simulink model "SingleInverterInfBus"  (R2020b)
settings: Solver=FixedStepAuto  StartTime=0.0  StopTime=20  FixedStep=Ts  RelTol=1e-3
values from neighbouring files (symbols this model uses):
  Cdc = 0.125    [Para.m]    (also in Para_VFM_FFL_Inverter.m = 0.101859163579; Para_VFM_FFL_Inverter_v2.m = 0.101859163579)
  Cf = 0.02    [Para.m]    (also in Para_VFM_FFL_Inverter.m; Para_VFM_FFL_Inverter_v2.m)
  Lc = 0.02    [Para.m]    (also in Para_VFM_FFL_Inverter.m; Para_VFM_FFL_Inverter_v2.m)
  Lf = 0.05    [Para.m]    (also in Para_VFM_FFL_Inverter.m; Para_VFM_FFL_Inverter_v2.m)
  m = 5/100    (= 0.05)    [Para.m]    (also in Para_VFM_FFL_Inverter.m; Para_VFM_FFL_Inverter_v2.m)
  Rline = Xline/5    (= 0.19)    [Para.m]    (also in Para_VFM_FFL_Inverter.m; Para_VFM_FFL_Inverter_v2.m)
  Sbase = 1    [Para.m]    (also in Para_VFM_FFL_Inverter.m; Para_VFM_FFL_Inverter_v2.m)
  Ts = 1/Fs    (= 0.0001)    [Para.m]    (also in Para_VFM_FFL_Inverter.m; Para_VFM_FFL_Inverter_v2.m = 5e-05)
  Vbase = 1    [Para.m]    (also in Para_VFM_FFL_Inverter.m; Para_VFM_FFL_Inverter_v2.m)
  vdc_ref = 2.5    [Para.m]    (also in Para_VFM_FFL_Inverter.m; Para_VFM_FFL_Inverter_v2.m)
  w_droop = 1*2*pi    (= 6.28318530718)    [Para.m]    (also in Para_VFM_FFL_Inverter.m = 31.4159265359; Para_VFM_FFL_Inverter_v2.m = 31.4159265359)
  w_i = 600*2*pi    (= 3769.91118431)    [Para.m]    (also in Para_VFM_FFL_Inverter.m; Para_VFM_FFL_Inverter_v2.m)
  w_pll = 15*2*pi    (= 94.2477796077)    [Para.m]    (also in Para_VFM_FFL_Inverter.m; Para_VFM_FFL_Inverter_v2.m)
  w_tau = 200*2*pi    (= 1256.63706144)    [Para.m]    (also in Para_VFM_FFL_Inverter.m; Para_VFM_FFL_Inverter_v2.m)
  w_v = 300*2*pi    (= 1884.95559215)    [Para.m]    (also in Para_VFM_FFL_Inverter.m; Para_VFM_FFL_Inverter_v2.m)
  w_vdc = 5*2*pi    (= 31.4159265359)    [Para.m]    (also in Para_VFM_FFL_Inverter.m; Para_VFM_FFL_Inverter_v2.m)
  Wbase = 2*pi*50    (= 314.159265359)    [Para.m]    (also in Para_VFM_FFL_Inverter.m; Para_VFM_FFL_Inverter_v2.m)
  Xline = 0.95    [Para.m]    (also in Para_VFM_FFL_Inverter.m; Para_VFM_FFL_Inverter_v2.m)
  Zbase = Vbase/Ibase    (= 1)    [Para.m]    (also in Para_VFM_FFL_Inverter.m; Para_VFM_FFL_Inverter_v2.m)
undefined symbols (not defined in the file or in its folder): DiscIntNeverNeededParam, initial
libraries: powerlib x282, SimplusGT x7
(part 1 of 8)
settings Model: Creator=admin_user  LastModifiedBy=admin_user
settings DataIOCC: ReturnWorkspaceOutputs=off

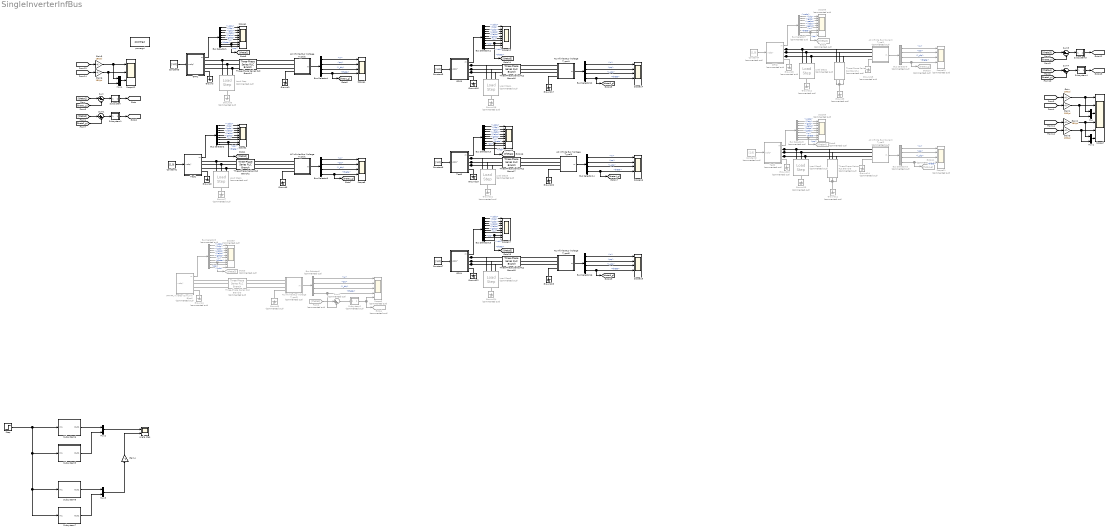
== system SingleInverterInfBus ==
  AC Infinite Bus (Current Type)1 : Subsystem  Commented=on  AncestorBlock=|  mask{Ts=Ts, Sbase=Sbase, Vbase=Vbase, Wbase=Wbase, id=1, iq=0, theta0=0, w=1}
      | SimplusGT/AC Infinite Bus
      | (Current Type)
      mask prompts: Ts "Ts (s), sampling period"; Sbase "Sbase (VA), base power"; Vbase "Vbase (V), base voltage"; Wbase "Wbase (rad/s), base angular frequency"; id "id (pu), d-axis current"; iq "iq (pu), q-axis current"; theta0 "theta0 (rad), initial angle"; w "w (pu), angular frequency"
  AC Infinite Bus (Current Type)2 : Subsystem  Commented=on  AncestorBlock=|  mask{Ts=Ts, Sbase=Sbase, Vbase=Vbase, Wbase=Wbase, id=1, iq=0, theta0=0, w=1}
      | SimplusGT/AC Infinite Bus
      | (Current Type)
      mask prompts: Ts "Ts (s), sampling period"; Sbase "Sbase (VA), base power"; Vbase "Vbase (V), base voltage"; Wbase "Wbase (rad/s), base angular frequency"; id "id (pu), d-axis current"; iq "iq (pu), q-axis current"; theta0 "theta0 (rad), initial angle"; w "w (pu), angular frequency"
  AC Infinite Bus (Voltage Type)1 : Subsystem  AncestorBlock=|  mask{Ts=Ts, Sbase=Sbase, Vbase=Vbase, Wbase=Wbase, vd=1, vq=0, theta0=0, w=Wbase*1, R=1e-30}
      | SimplusGT/AC Infinite Bus
      | (Voltage Type)
      mask prompts: Ts "Ts (s), samping period"; Sbase "Sbase (VA), power base"; Vbase "Vbase (V), voltage base"; Wbase "Wbase (rad/s), frequency base"; vd "vd (pu), d-axis voltage"; vq "vq (pu), q-axis voltage"; theta0 "theta0 (rad), initial angle"; w "w (rad/s), frequency"; R "R (Ohm), resistance"
  AC Infinite Bus (Voltage Type)2 : Subsystem  AncestorBlock=|  mask{Ts=Ts, Sbase=Sbase, Vbase=Vbase, Wbase=Wbase, vd=1, vq=0, theta0=0, w=Wbase*1, R=1e-30}
      | SimplusGT/AC Infinite Bus
      | (Voltage Type)
      mask prompts: Ts "Ts (s), samping period"; Sbase "Sbase (VA), power base"; Vbase "Vbase (V), voltage base"; Wbase "Wbase (rad/s), frequency base"; vd "vd (pu), d-axis voltage"; vq "vq (pu), q-axis voltage"; theta0 "theta0 (rad), initial angle"; w "w (rad/s), frequency"; R "R (Ohm), resistance"
  AC Infinite Bus (Voltage Type)3 : Subsystem  Commented=on  AncestorBlock=|  mask{Ts=Ts, Sbase=Sbase, Vbase=Vbase, Wbase=Wbase, vd=1, vq=0, theta0=0, w=Wbase*1, R=1e-30}
      | SimplusGT/AC Infinite Bus
      | (Voltage Type)
      mask prompts: Ts "Ts (s), samping period"; Sbase "Sbase (VA), power base"; Vbase "Vbase (V), voltage base"; Wbase "Wbase (rad/s), frequency base"; vd "vd (pu), d-axis voltage"; vq "vq (pu), q-axis voltage"; theta0 "theta0 (rad), initial angle"; w "w (rad/s), frequency"; R "R (Ohm), resistance"
  AC Infinite Bus (Voltage Type)4 : Subsystem  AncestorBlock=|  mask{Ts=Ts, Sbase=Sbase, Vbase=Vbase, Wbase=Wbase, vd=1, vq=0, theta0=0, w=Wbase*1, R=1e-30}
      | SimplusGT/AC Infinite Bus
      | (Voltage Type)
      mask prompts: Ts "Ts (s), samping period"; Sbase "Sbase (VA), power base"; Vbase "Vbase (V), voltage base"; Wbase "Wbase (rad/s), frequency base"; vd "vd (pu), d-axis voltage"; vq "vq (pu), q-axis voltage"; theta0 "theta0 (rad), initial angle"; w "w (rad/s), frequency"; R "R (Ohm), resistance"
  AC Infinite Bus (Voltage Type)5 : Subsystem  AncestorBlock=|  mask{Ts=Ts, Sbase=Sbase, Vbase=Vbase, Wbase=Wbase, vd=1, vq=0, theta0=0, w=Wbase*1, R=1e-30}
      | SimplusGT/AC Infinite Bus
      | (Voltage Type)
      mask prompts: Ts "Ts (s), samping period"; Sbase "Sbase (VA), power base"; Vbase "Vbase (V), voltage base"; Wbase "Wbase (rad/s), frequency base"; vd "vd (pu), d-axis voltage"; vq "vq (pu), q-axis voltage"; theta0 "theta0 (rad), initial angle"; w "w (rad/s), frequency"; R "R (Ohm), resistance"
  AC Infinite Bus (Voltage Type)6 : Subsystem  AncestorBlock=|  mask{Ts=Ts, Sbase=Sbase, Vbase=Vbase, Wbase=Wbase, vd=1, vq=0, theta0=0, w=Wbase*1, R=1e-30}
      | SimplusGT/AC Infinite Bus
      | (Voltage Type)
      mask prompts: Ts "Ts (s), samping period"; Sbase "Sbase (VA), power base"; Vbase "Vbase (V), voltage base"; Wbase "Wbase (rad/s), frequency base"; vd "vd (pu), d-axis voltage"; vq "vq (pu), q-axis voltage"; theta0 "theta0 (rad), initial angle"; w "w (rad/s), frequency"; R "R (Ohm), resistance"
  Angle step : Scope  NumInputPorts=2
  Bus Selector1 : BusSelector  OutputSignals=vcdq,ildq,igdq,vcabc,ilabc,igabc,w,theta,pq
  Bus Selector10 : BusSelector  Commented=on  OutputSignals=w,pq,i_dq,theta
  Bus Selector11 : BusSelector  OutputSignals=vcdq,ildq,igdq,vcabc,ilabc,igabc,w,theta,pq,vdc
  Bus Selector{4..5,12,14,16} (5 alike) : BusSelector  OutputSignals=w,pq,i_dq,theta
  Bus Selector13 : BusSelector  OutputSignals=vcdq,ildq,igdq,vcabc,ilabc,igabc,w,theta,pq,vdc
  Bus Selector15 : BusSelector  OutputSignals=vcdq,ildq,igdq,vcabc,ilabc,igabc,w,theta,pq,vdc
  Bus Selector2 : BusSelector  OutputSignals=vcdq,ildq,igdq,vcabc,ilabc,igabc,w,theta,pq
  Bus Selector3 : BusSelector  Commented=on  OutputSignals=vcdq,ildq,igdq,vcabc,ilabc,igabc,w,theta,pq,vdc
  Bus Selector6 : BusSelector  Commented=on  OutputSignals=w,pq,i_dq,theta
  Bus Selector7 : BusSelector  Commented=on  OutputSignals=vcdq,ildq,igdq,vcabc,ilabc,igabc,w,theta,pq
  Bus Selector8 : BusSelector  Commented=on  OutputSignals=vcdq,ildq,igdq,vcabc,ilabc,igabc,w,theta,pq
  Bus Selector9 : BusSelector  Commented=on  OutputSignals=w,pq,i_dq,theta
  Constant{1,3,5..7} (5 alike) : Constant  Value=[1,0]
  Constant2 : Constant  Commented=on  Value=[1,0]
  Constant4 : Constant  Commented=on  Value=[1,0]
  From2 : From  Commented=on  GotoTag=theta3
  GFM1 : Subsystem  mask{Ts=Ts, Sbase=Sbase, Vbase=Vbase, Wbase=Wbase, w_i=w_i, w_v=w_v, w_droop=w_droop, m=m, Lf=Lf, Cf=Cf, Lc=Lc}
      mask prompts: Ts "Ts (s), sampling period"; Sbase "Sbase (VA), base power"; Vbase "Vbase (V), base voltage"; Wbase "Wbase (rad/s), base frequency"; w_i "w_i (rad/s), current-loop bandwidth"; w_v "w_v (rad/s), voltage-loop bandwidth"; w_droop "w_droop (rad/s), droop bandwidth"; m "m (pu), frequency droop gain"; Lf "Lf (pu), LCL filter"; Cf "Cf (pu), LCL filter"; Lc "Lc (pu), LCL filter"
  GFM2 : Subsystem  Commented=on  mask{Ts=Ts, Sbase=Sbase, Vbase=Vbase, Wbase=Wbase, w_i=w_i, w_v=w_v, w_droop=w_droop, m=m, Lf=Lf, Cf=Cf, Lc=Lc}
      mask prompts: Ts "Ts (s), sampling period"; Sbase "Sbase (VA), base power"; Vbase "Vbase (V), base voltage"; Wbase "Wbase (rad/s), base frequency"; w_i "w_i (rad/s), current-loop bandwidth"; w_v "w_v (rad/s), voltage-loop bandwidth"; w_droop "w_droop (rad/s), droop bandwidth"; m "m (pu), frequency droop gain"; Lf "Lf (pu), LCL filter"; Cf "Cf (pu), LCL filter"; Lc "Lc (pu), LCL filter"
  GFM3 : Subsystem  mask{Ts=Ts, Sbase=Sbase, Vbase=Vbase, Wbase=Wbase, w_i=w_i, w_v=w_v, w_droop=w_droop, m=m, Lf=Lf, Cf=Cf, Lc=Lc, Cdc=Cdc, vdc_ref=vdc_ref, w_vdc=w_vdc/10}
      mask prompts: Ts "Ts (s), sampling period"; Sbase "Sbase (VA), base power"; Vbase "Vbase (V), base voltage"; Wbase "Wbase (rad/s), base frequency"; w_i "w_i (rad/s), current-loop bandwidth"; w_v "w_v (rad/s), voltage-loop bandwidth"; w_droop "w_droop (rad/s), droop bandwidth"; m "m (pu), frequency droop gain"; Lf "Lf (pu), LCL filter"; Cf "Cf (pu), LCL filter"; Lc "Lc (pu), LCL filter"
  GFM4 : Subsystem  mask{Ts=Ts, Sbase=Sbase, Vbase=Vbase, Wbase=Wbase, w_i=w_i, w_v=w_v, w_droop=w_droop, m=m, Lf=Lf, Cf=Cf, Lc=Lc, Cdc=Cdc, vdc_ref=vdc_ref, w_vdc=w_vdc/1}
      mask prompts: Ts "Ts (s), sampling period"; Sbase "Sbase (VA), base power"; Vbase "Vbase (V), base voltage"; Wbase "Wbase (rad/s), base frequency"; w_i "w_i (rad/s), current-loop bandwidth"; w_v "w_v (rad/s), voltage-loop bandwidth"; w_droop "w_droop (rad/s), droop bandwidth"; m "m (pu), frequency droop gain"; Lf "Lf (pu), LCL filter"; Cf "Cf (pu), LCL filter"; Lc "Lc (pu), LCL filter"
  Gain{,1..3,5..6} (6 alike) : Gain  Gain=180/pi
  Gain4 : Gain  Gain=-1
  Goto10 : Goto  Commented=on  GotoTag=theta3_g
  Goto11 : Goto  Commented=on  GotoTag=theta4_g
  Goto3 : Goto  Commented=on  GotoTag=theta3
  Goto4 : Goto  Commented=on  GotoTag=theta_diff3
  Goto8 : Goto  Commented=on  GotoTag=theta4
  Goto9 : Goto  Commented=on  GotoTag=theta3
  Ground{,1..3,16..17,19..20,22..23} (10 alike) : powerlib/Elements/Ground  LConnTagsString=a
  Ground{4..15,18,21,24} (15 alike) : powerlib/Elements/Ground  Commented=on  LConnTagsString=a
  Load Step{,1,4..6} (5 alike) : SimplusGT/Load Step  Commented=on  t0=0  R=4*Zbase  Reverse=0
      settings: SourceProductName=Simplus Grid Tool
  Load Step2 : SimplusGT/Load Step  Commented=on  t0=0  R=3*Zbase  Reverse=0
      settings: SourceProductName=Simplus Grid Tool
  Load Step3 : SimplusGT/Load Step  Commented=on  t0=0  R=3*Zbase  Reverse=0
      settings: SourceProductName=Simplus Grid Tool
  Mux{,1..4} (5 alike) : Mux  Inputs=2
  Scope1 : Scope  NumInputPorts=9
  Scope10 : Scope  Commented=on  NumInputPorts=5
  Scope11 : Scope  Commented=on  NumInputPorts=5
  Scope12 : Scope  NumInputPorts=3
  Scope13 : Scope  NumInputPorts=10
  Scope{4..5,14,16,18} (5 alike) : Scope  NumInputPorts=5
  Scope15 : Scope  NumInputPorts=10
  Scope17 : Scope  NumInputPorts=10
  Scope2 : Scope  NumInputPorts=9
  Scope3 : Scope  Commented=on  NumInputPorts=10
  Scope6 : Scope  Commented=on  NumInputPorts=5
  Scope7 : Scope  NumInputPorts=6
  Scope8 : Scope  Commented=on  NumInputPorts=9
  Scope9 : Scope  Commented=on  NumInputPorts=9
  Step : Step  Time=3  After=-1  SampleTime=0
  Subsystem : Subsystem
  Subsystem1 : Subsystem
  Subsystem2 : Subsystem  Commented=on
  Subsystem3 : Subsystem
  Subsystem4 : Subsystem
  Subsystem5 : Subsystem  mask{kp=1*2*pi, ki=1*2*pi*2.5*2*pi}
  Subsystem6 : Subsystem  mask{kd=1/(2.5*2*pi), ki=1*2*pi*2.5*2*pi}
  Subsystem7 : Subsystem  mask{kp=1*2*pi, ki=1*2*pi*2.5*2*pi}
  Subsystem8 : Subsystem  mask{kd=1/(2.5*2*pi), ki=1*2*pi*2.5*2*pi}
  Sum{,1,3..4} (4 alike) : Sum  Inputs=|+-
  Sum2 : Sum  Commented=on  Inputs=|+-
  Test1 : Subsystem  mask{Ts=Ts, Sbase=Sbase, Vbase=Vbase, Wbase=Wbase, w_i=w_i*1, w_v=w_v, w_pll=w_pll, w_tau=w_tau, m=m, Lf=Lf, Cf=Cf, Lc=Lc}
      mask prompts: Ts "Ts (s), sampling period"; Sbase "Sbase (VA), base power"; Vbase "Vbase (V), base voltage"; Wbase "Wbase (rad/s), base frequency"; w_i "w_i (rad/s), current-loop bandwidth"; w_v "w_v (rad/s), voltage-loop bandwidth"; w_pll "w_pll (rad/s), PLL bandwidth"; w_tau "w_tau (rad/s), pll LPF bandwidth"; m "m (pu), frequency droop gain"; Lf "Lf (pu), LCL filter"; Cf "Cf (pu), LCL filter"; Lc "Lc (pu), LCL filter"
  Test2 : Subsystem  Commented=on  mask{Ts=Ts, Sbase=Sbase, Vbase=Vbase, Wbase=Wbase, w_i=w_i, w_v=w_v, w_pll=w_pll, w_tau=w_tau, m=m, Lf=Lf, Cf=Cf, Lc=Lc}
      mask prompts: Ts "Ts (s), sampling period"; Sbase "Sbase (VA), base power"; Vbase "Vbase (V), base voltage"; Wbase "Wbase (rad/s), base frequency"; w_i "w_i (rad/s), current-loop bandwidth"; w_v "w_v (rad/s), voltage-loop bandwidth"; w_pll "w_pll (rad/s), PLL bandwidth"; w_tau "w_tau (rad/s), pll LPF bandwidth"; m "m (pu), frequency droop gain"; Lf "Lf (pu), LCL filter"; Cf "Cf (pu), LCL filter"; Lc "Lc (pu), LCL filter"
  Test3 : Subsystem  mask{Ts=Ts, Sbase=Sbase, Vbase=Vbase, Wbase=Wbase, w_i=w_i*1, w_v=w_v, w_pll=w_pll, w_tau=w_tau, m=m, Lf=Lf, Cf=Cf, Lc=Lc, Cdc=Cdc, vdc_ref=vdc_ref, w_vdc=w_vdc/10}
      mask prompts: Ts "Ts (s), sampling period"; Sbase "Sbase (VA), base power"; Vbase "Vbase (V), base voltage"; Wbase "Wbase (rad/s), base frequency"; w_i "w_i (rad/s), current-loop bandwidth"; w_v "w_v (rad/s), voltage-loop bandwidth"; w_pll "w_pll (rad/s), PLL bandwidth"; w_tau "w_tau (rad/s), pll LPF bandwidth"; m "m (pu), frequency droop gain"; Lf "Lf (pu), LCL filter"; Cf "Cf (pu), LCL filter"; Lc "Lc (pu), LCL filter"
  Three-Phase Series RLC Branch{1..2,6..8} (5 alike) : powerlib/Elements/Three-Phase Series RLC Branch  LConnTagsString=A|B|C  RConnTagsString=A|B|C  BranchType=RL  Resistance=Rline*Zbase  Inductance=Xline*Zbase/Wbase  Capacitance=1/Wbase  Measurements=None
  Three-Phase Series RLC Branch3 : powerlib/Elements/Three-Phase Series RLC Branch  Commented=on  LConnTagsString=A|B|C  RConnTagsString=A|B|C  BranchType=RL  Resistance=Rline*Zbase  Inductance=Xline*Zbase/Wbase  Capacitance=1/Wbase  Measurements=None
  Three-Phase Series RLC Branch4 : powerlib/Elements/Three-Phase Series RLC Branch  Commented=on  LConnTagsString=A|B|C  RConnTagsString=A|B|C  BranchType=RL  Resistance=Rline*Zbase  Inductance=Xline*Zbase/Wbase  Capacitance=1/Wbase  Measurements=None
  Three-Phase Series RLC Branch5 : powerlib/Elements/Three-Phase Series RLC Branch  Commented=on  LConnTagsString=A|B|C  RConnTagsString=A|B|C  BranchType=RL  Resistance=Rline*Zbase  Inductance=Xline*Zbase/Wbase  Capacitance=1/Wbase  Measurements=None
  VFM-FFL Inverter (Simulink Block) : Subsystem  Commented=on  mask{Ts=Ts, Sbase=Sbase, Vbase=Vbase, Wbase=Wbase, w_i=w_i, w_v=w_v, w_pll=w_pll, w_tau=w_tau, m=m, wLf=Lf, wCf=Cf, wLc=Lc, Cdc=Cdc, vdc_ref=vdc_ref, w_vdc=w_vdc}
      mask prompts: Ts "Ts (s), sampling period"; Sbase "Sbase (VA), base power"; Vbase "Vbase (V), base voltage"; Wbase "Wbase (rad/s), base frequency"; w_i "w_i (rad/s), current-loop bandwidth"; w_v "w_v (rad/s), voltage-loop bandwidth"; w_pll "w_pll (rad/s), PLL bandwidth"; w_tau "w_tau (rad/s), pll LPF bandwidth"; m "m (pu), frequency droop gain"; wLf "wLf (pu), LCL filter"; wCf "wCf (pu), LCL filter"; wLc "wLc (pu), LCL filter"; Cdc "Cdc (pu), dc-link capacitor"; vdc_ref "vdc_ref (pu), dc-link voltage reference"; w_vdc "w_vdc (rad/s), dc-link voltage loop bandwidth"
  powergui : powerlib/powergui  Priority=1  SimulationMode=Discrete  SampleTime=Ts  frequency=60  Iterations=50  frequencyindice=0  Pbase=100e6  ErrMax=1e-4  UnitsV=kV  UnitsW=MW  buscounter=0  FunctionMessages=off  echomessages=off  EnableUseOfTLC=off  CurrentSourceSwitches=off  DisableSnubberDevices=off  DisableRonSwitches=off  DisableVfSwitches=off  DisplayEquations=off  AutomaticDiscreteSolvers=off  SolverType=Tustin/Backward Euler (TBE)  Interpol=off  ExternalGateDelay=off  methode=off  Ts=100  x0status=blocks  SPID=on  SwTol=0  HookPort=off  NonlinearTolerance=1e-4  nMaxIteration=100  ContinueOnMaxIteration=off  RestoreLinks=warning  ResistiveCurrentMeasurement=off  Frange=[0:2:500]  Ylog=off  Xlog=on  ShowGrid=off  save=off  variable=ZData  structure=0  ZoomFFT=off  StartTime=0.0  cycles=1  DisplayStyle=1  fundamental=60  FreqAxis=off  MaxFrequency=1000  frequencyindicesteady=1  RmsSteady=1  display=off
  wires:
  Constant3/1 -> GFM1/1(vcdq*)
  Bus Selector1/7 -> Scope1/7  "<w>"
  Bus Selector1/3 -> Scope1/3  "<igdq>"
  Bus Selector1/2 -> Scope1/2  "<ildq>"
  Bus Selector1/1 -> Scope1/1  "<vcdq>"
  Bus Selector1/5 -> Scope1/5  "<ilabc>"
  Bus Selector1/6 -> Scope1/6  "<igabc>"
  Bus Selector1/4 -> Scope1/4  "<vcabc>"
  Bus Selector1/8 -> [theta1], Scope1/8  "<theta>"
  GFM1/1(m) -> Bus Selector1/1
  Test1/1(m) -> Bus Selector2/1
  Bus Selector2/8 -> Scope2/8, [theta2]  "<theta>"
  Bus Selector2/6 -> Scope2/6  "<igabc>"
  Bus Selector2/1 -> Scope2/1  "<vcdq>"
  Bus Selector2/2 -> Scope2/2  "<ildq>"
  Bus Selector2/5 -> Scope2/5  "<ilabc>"
  Bus Selector2/4 -> Scope2/4  "<vcabc>"
  Bus Selector2/3 -> Scope2/3  "<igdq>"
  Bus Selector2/7 -> Scope2/7  "<w>"
  Constant1/1 -> Test1/1(vcdq*)
  Bus Selector3/5 -> Scope3/5  "<ilabc>"
  Bus Selector3/2 -> Scope3/2  "<ildq>"
  Bus Selector3/1 -> Scope3/1  "<vcdq>"
  Bus Selector3/6 -> Scope3/6  "<igabc>"
  Bus Selector3/4 -> Scope3/4  "<vcabc>"
  Bus Selector3/7 -> Scope3/7  "<w>"
  Bus Selector3/8 -> Scope3/8, Goto3/1  "<theta>"
  Bus Selector3/3 -> Scope3/3  "<igdq>"
  VFM-FFL Inverter (Simulink Block)/1(m) -> Bus Selector3/1
  AC Infinite Bus (Voltage Type)2/1(m) -> Bus Selector4/1
  Bus Selector4/1 -> Scope4/1  "<w>"
  Bus Selector4/2 -> Scope4/2  "<pq>"
  Bus Selector4/3 -> Scope4/3  "<i_dq>"
  Bus Selector4/4 -> Scope4/4, [theta1_g]  "<theta>"
  [theta1] -> Sum/1
  Bus Selector5/3 -> Scope5/3  "<i_dq>"
  Bus Selector5/4 -> [theta2_g], Scope5/4  "<theta>"
  Bus Selector5/2 -> Scope5/2  "<pq>"
  AC Infinite Bus (Voltage Type)1/1(m) -> Bus Selector5/1
  Bus Selector5/1 -> Scope5/1  "<w>"
  [theta2] -> Sum1/1
  Bus Selector6/2 -> Scope6/2  "<pq>"
  From2/1 -> Sum2/1
  AC Infinite Bus (Voltage Type)3/1(m) -> Bus Selector6/1
  Bus Selector6/4 -> Scope6/4, Sum2/2  "<theta>"
  Bus Selector6/1 -> Scope6/1  "<w>"
  Bus Selector6/3 -> Scope6/3  "<i_dq>"
  Sum/1 -> Subsystem/1(In1)
  Sum1/1 -> Subsystem1/1(In1)
  Subsystem1/1(Out1) -> [theta_diff2]
  Sum2/1 -> Subsystem2/1(In1)
  Subsystem2/1(Out1) -> Goto4/1, Scope6/5
  [theta_diff1] -> Gain/1
  [theta_diff2] -> Gain1/1
  Subsystem/1(Out1) -> [theta_diff1]
  Bus Selector1/9 -> Scope1/9  "<pq>"
  Bus Selector2/9 -> Scope2/9  "<pq>"
  Bus Selector3/9 -> Scope3/9  "<pq>"
  Bus Selector3/10 -> Scope3/10  "<vdc>"
  Gain/1 -> Scope7/1, Mux/1
  Gain1/1 -> Mux/2, Scope7/2
  [theta1_g] -> Sum/2
  [theta2_g] -> Sum1/2
  Bus Selector8/9 -> Scope9/9  "<pq>"
  Bus Selector7/9 -> Scope8/9  "<pq>"
  Bus Selector10/3 -> Scope11/3  "<i_dq>"
  Bus Selector10/1 -> Scope11/1  "<w>"
  AC Infinite Bus (Current Type)1/1(m) -> Bus Selector9/1
  AC Infinite Bus (Current Type)2/1(m) -> Bus Selector10/1
  Test2/1(m) -> Bus Selector8/1
  Bus Selector8/1 -> Scope9/1  "<vcdq>"
  Bus Selector9/1 -> Scope10/1  "<w>"
  Bus Selector8/3 -> Scope9/3  "<igdq>"
  Constant2/1 -> Test2/1(vcdq*)
  Bus Selector7/6 -> Scope8/6  "<igabc>"
  Bus Selector8/7 -> Scope9/7  "<w>"
  Bus Selector8/2 -> Scope9/2  "<ildq>"
  Bus Selector8/8 -> Scope9/8, Goto8/1  "<theta>"
  Bus Selector7/8 -> Goto9/1, Scope8/8  "<theta>"
  Bus Selector8/5 -> Scope9/5  "<ilabc>"
  Bus Selector9/4 -> Scope10/4, Goto10/1  "<theta>"
  Bus Selector7/1 -> Scope8/1  "<vcdq>"
  Bus Selector8/4 -> Scope9/4  "<vcabc>"
  Bus Selector7/4 -> Scope8/4  "<vcabc>"
  Constant4/1 -> GFM2/1(vcdq*)
  Bus Selector7/5 -> Scope8/5  "<ilabc>"
  Bus Selector7/3 -> Scope8/3  "<igdq>"
  Bus Selector9/2 -> Scope10/2  "<pq>"
  Bus Selector10/4 -> Goto11/1, Scope11/4  "<theta>"
  Bus Selector7/7 -> Scope8/7  "<w>"
  Bus Selector8/6 -> Scope9/6  "<igabc>"
  GFM2/1(m) -> Bus Selector7/1
  Bus Selector10/2 -> Scope11/2  "<pq>"
  Bus Selector7/2 -> Scope8/2  "<ildq>"
  Bus Selector9/3 -> Scope10/3  "<i_dq>"
  [theta3_g] -> Sum3/2
  Subsystem3/1(Out1) -> [theta_diff3]
  [theta4_g] -> Sum4/2
  Sum3/1 -> Subsystem3/1(In1)
  Subsystem4/1(Out1) -> [theta_diff4]
  Sum4/1 -> Subsystem4/1(In1)
  [theta3] -> Sum3/1
  [theta4] -> Sum4/1
  [theta_diff4] -> Gain3/1
  [theta_diff3] -> Gain2/1
  Mux/1 -> Scope7/3
  Gain2/1 -> Mux1/1, Scope7/4
  Gain3/1 -> Mux1/2, Scope7/5
  Mux1/1 -> Scope7/6
  Mux2/1 -> Angle step/1
  Subsystem6/1(Out1) -> Mux2/1
  Subsystem5/1(Out1) -> Mux2/2
  Subsystem7/1(Out1) -> Mux3/2
  Step/1 -> Subsystem7/1(In1), Subsystem8/1(In1), Subsystem5/1(In1), Subsystem6/1(In1)
  Subsystem8/1(Out1) -> Mux3/1
  Gain4/1 -> Angle step/2
  Mux3/1 -> Gain4/1
  [theta_diff2] -> Gain6/1
  [theta_diff1] -> Gain5/1
  Gain6/1 -> Scope12/2, Mux4/2
  Gain5/1 -> Scope12/1, Mux4/1
  Mux4/1 -> Scope12/3
  Bus Selector11/9 -> Scope13/9  "<pq>"
  AC Infinite Bus (Voltage Type)4/1(m) -> Bus Selector12/1
  Bus Selector12/1 -> Scope14/1  "<w>"
  Bus Selector11/6 -> Scope13/6  "<igabc>"
  Bus Selector11/5 -> Scope13/5  "<ilabc>"
  Bus Selector11/8 -> [theta3], Scope13/8  "<theta>"
  Bus Selector12/4 -> Scope14/4, [theta3_g]  "<theta>"
  Bus Selector11/1 -> Scope13/1  "<vcdq>"
  GFM3/1(m) -> Bus Selector11/1
  Bus Selector12/2 -> Scope14/2  "<pq>"
  Bus Selector11/3 -> Scope13/3  "<igdq>"
  Bus Selector11/4 -> Scope13/4  "<vcabc>"
  Constant5/1 -> GFM3/1(vcdq*)
  Bus Selector11/7 -> Scope13/7  "<w>"
  Bus Selector11/2 -> Scope13/2  "<ildq>"
  Bus Selector12/3 -> Scope14/3  "<i_dq>"
  AC Infinite Bus (Voltage Type)5/1(m) -> Bus Selector14/1
  Bus Selector13/9 -> Scope15/9  "<pq>"
  Bus Selector14/3 -> Scope16/3  "<i_dq>"
  Bus Selector14/1 -> Scope16/1  "<w>"
  Bus Selector14/4 -> [theta4_g], Scope16/4  "<theta>"
  Test3/1(m) -> Bus Selector13/1
  Bus Selector13/1 -> Scope15/1  "<vcdq>"
  Bus Selector13/3 -> Scope15/3  "<igdq>"
  Bus Selector13/4 -> Scope15/4  "<vcabc>"
  Constant6/1 -> Test3/1(vcdq*)
  Bus Selector13/7 -> Scope15/7  "<w>"
  Bus Selector13/2 -> Scope15/2  "<ildq>"
  Bus Selector13/8 -> Scope15/8, [theta4]  "<theta>"
  Bus Selector13/5 -> Scope15/5  "<ilabc>"
  Bus Selector14/2 -> Scope16/2  "<pq>"
  Bus Selector13/6 -> Scope15/6  "<igabc>"
  Bus Selector11/10 -> Scope13/10  "<vdc>"
  Bus Selector13/10 -> Scope15/10  "<vdc>"
  Bus Selector15/10 -> Scope17/10  "<vdc>"
  Bus Selector16/3 -> Scope18/3  "<i_dq>"
  Bus Selector15/2 -> Scope17/2  "<ildq>"
  Constant7/1 -> GFM4/1(vcdq*)
  Bus Selector15/3 -> Scope17/3  "<igdq>"
  Bus Selector15/7 -> Scope17/7  "<w>"
  GFM4/1(m) -> Bus Selector15/1
  Bus Selector15/8 -> [theta5], Scope17/8  "<theta>"
  Bus Selector16/4 -> Scope18/4, [theta5_g]  "<theta>"
  Bus Selector15/6 -> Scope17/6  "<igabc>"
  Bus Selector16/1 -> Scope18/1  "<w>"
  Bus Selector15/9 -> Scope17/9  "<pq>"
  Bus Selector15/5 -> Scope17/5  "<ilabc>"
  AC Infinite Bus (Voltage Type)6/1(m) -> Bus Selector16/1
  Bus Selector15/4 -> Scope17/4  "<vcabc>"
  Bus Selector16/2 -> Scope18/2  "<pq>"
  Bus Selector15/1 -> Scope17/1  "<vcdq>"
  connections:
  Three-Phase Series RLC Branch1/RConn1 -- Load Step/LConn1 -- GFM1/RConn1
  Three-Phase Series RLC Branch1/RConn3 -- Load Step/LConn3 -- GFM1/RConn3
  Three-Phase Series RLC Branch1/RConn2 -- Load Step/LConn2 -- GFM1/RConn2
  AC Infinite Bus (Voltage Type)2/LConn1 -- Three-Phase Series RLC Branch1/LConn1
  AC Infinite Bus (Voltage Type)2/LConn2 -- Three-Phase Series RLC Branch1/LConn2
  AC Infinite Bus (Voltage Type)2/LConn3 -- Three-Phase Series RLC Branch1/LConn3
  Ground/LConn1 -- GFM1/RConn4
  AC Infinite Bus (Voltage Type)2/LConn4 -- Ground1/LConn1
  Three-Phase Series RLC Branch2/RConn2 -- Load Step1/LConn2 -- Test1/RConn2
  AC Infinite Bus (Voltage Type)1/LConn1 -- Three-Phase Series RLC Branch2/LConn1
  AC Infinite Bus (Voltage Type)1/LConn4 -- Ground3/LConn1
  Ground2/LConn1 -- Test1/RConn4
  Three-Phase Series RLC Branch2/RConn1 -- Load Step1/LConn1 -- Test1/RConn1
  AC Infinite Bus (Voltage Type)1/LConn2 -- Three-Phase Series RLC Branch2/LConn2
  AC Infinite Bus (Voltage Type)1/LConn3 -- Three-Phase Series RLC Branch2/LConn3
  Three-Phase Series RLC Branch2/RConn3 -- Load Step1/LConn3 -- Test1/RConn3
  AC Infinite Bus (Voltage Type)3/LConn3 -- Three-Phase Series RLC Branch3/LConn3
  AC Infinite Bus (Voltage Type)3/LConn2 -- Three-Phase Series RLC Branch3/LConn2
  AC Infinite Bus (Voltage Type)3/LConn1 -- Three-Phase Series RLC Branch3/LConn1
  Three-Phase Series RLC Branch3/RConn1 -- VFM-FFL Inverter (Simulink Block)/RConn1
  Three-Phase Series RLC Branch3/RConn3 -- VFM-FFL Inverter (Simulink Block)/RConn3
  Three-Phase Series RLC Branch3/RConn2 -- VFM-FFL Inverter (Simulink Block)/RConn2
  AC Infinite Bus (Voltage Type)3/LConn4 -- Ground5/LConn1
  Ground4/LConn1 -- VFM-FFL Inverter (Simulink Block)/RConn4
  Ground6/LConn1 -- Load Step/RConn1
  Ground7/LConn1 -- Load Step1/RConn1
  Test2/RConn3 -- AC Infinite Bus (Current Type)2/LConn3 -- Three-Phase Series RLC Branch5/RConn3 -- Load Step3/LConn3
  Test2/RConn2 -- AC Infinite Bus (Current Type)2/LConn2 -- Three-Phase Series RLC Branch5/RConn2 -- Load Step3/LConn2
  GFM2/RConn1 -- AC Infinite Bus (Current Type)1/LConn1 -- Three-Phase Series RLC Branch4/RConn1 -- Load Step2/LConn1
  GFM2/RConn3 -- AC Infinite Bus (Current Type)1/LConn3 -- Three-Phase Series RLC Branch4/RConn3 -- Load Step2/LConn3
  GFM2/RConn2 -- AC Infinite Bus (Current Type)1/LConn2 -- Three-Phase Series RLC Branch4/RConn2 -- Load Step2/LConn2
  Test2/RConn1 -- AC Infinite Bus (Current Type)2/LConn1 -- Three-Phase Series RLC Branch5/RConn1 -- Load Step3/LConn1
  Ground8/LConn1 -- GFM2/RConn4
  Ground10/LConn1 -- Test2/RConn4
  Ground13/LConn1 -- Load Step3/RConn1
  Ground12/LConn1 -- Load Step2/RConn1
  Ground9/LConn1 -- Three-Phase Series RLC Branch4/LConn3 -- Three-Phase Series RLC Branch4/LConn1 -- Three-Phase Series RLC Branch4/LConn2
  Three-Phase Series RLC Branch5/LConn2 -- Three-Phase Series RLC Branch5/LConn3 -- Three-Phase Series RLC Branch5/LConn1 -- Ground11/LConn1
  AC Infinite Bus (Current Type)2/LConn4 -- Ground14/LConn1
  Ground15/LConn1 -- AC Infinite Bus (Current Type)1/LConn4
  GFM3/RConn1 -- Three-Phase Series RLC Branch6/RConn1 -- Load Step4/LConn1
  GFM3/RConn3 -- Three-Phase Series RLC Branch6/RConn3 -- Load Step4/LConn3
  GFM3/RConn2 -- Three-Phase Series RLC Branch6/RConn2 -- Load Step4/LConn2
  AC Infinite Bus (Voltage Type)4/LConn2 -- Three-Phase Series RLC Branch6/LConn2
  AC Infinite Bus (Voltage Type)4/LConn3 -- Three-Phase Series RLC Branch6/LConn3
  AC Infinite Bus (Voltage Type)4/LConn4 -- Ground17/LConn1
  Ground18/LConn1 -- Load Step4/RConn1
  AC Infinite Bus (Voltage Type)4/LConn1 -- Three-Phase Series RLC Branch6/LConn1
  Ground16/LConn1 -- GFM3/RConn4
  Test3/RConn3 -- Three-Phase Series RLC Branch7/RConn3 -- Load Step5/LConn3
  Test3/RConn2 -- Three-Phase Series RLC Branch7/RConn2 -- Load Step5/LConn2
  Test3/RConn1 -- Three-Phase Series RLC Branch7/RConn1 -- Load Step5/LConn1
  AC Infinite Bus (Voltage Type)5/LConn4 -- Ground20/LConn1
  AC Infinite Bus (Voltage Type)5/LConn1 -- Three-Phase Series RLC Branch7/LConn1
  Ground21/LConn1 -- Load Step5/RConn1
  AC Infinite Bus (Voltage Type)5/LConn3 -- Three-Phase Series RLC Branch7/LConn3
  AC Infinite Bus (Voltage Type)5/LConn2 -- Three-Phase Series RLC Branch7/LConn2
  Ground19/LConn1 -- Test3/RConn4
  GFM4/RConn3 -- Three-Phase Series RLC Branch8/RConn3 -- Load Step6/LConn3
  GFM4/RConn2 -- Three-Phase Series RLC Branch8/RConn2 -- Load Step6/LConn2
  GFM4/RConn1 -- Three-Phase Series RLC Branch8/RConn1 -- Load Step6/LConn1
  AC Infinite Bus (Voltage Type)6/LConn3 -- Three-Phase Series RLC Branch8/LConn3
  Ground22/LConn1 -- GFM4/RConn4
  Ground24/LConn1 -- Load Step6/RConn1
  AC Infinite Bus (Voltage Type)6/LConn1 -- Three-Phase Series RLC Branch8/LConn1
  AC Infinite Bus (Voltage Type)6/LConn4 -- Ground23/LConn1
  AC Infinite Bus (Voltage Type)6/LConn2 -- Three-Phase Series RLC Branch8/LConn2

== system SingleInverterInfBus/AC Infinite Bus (Current Type)1 ==
  note: Electrical Circuit
  note: Auxiliary
  note: Current-type infinite bus.
      |
      | Author(s): Yitong Li
      |
      | Notes:
      |
      | Current-type means the infinite bus is a current source rather than a voltage source.
      |
      | The system is in source convention.
  Bus Creator : BusCreator  Inputs=7
  Constant : Constant  Value=[id iq]
  Constant1 : Constant  Value=w
  Constant2 : Constant  Value=theta0
  Constant3 : Constant  Value=2*pi
  Controlled Current Source : powerlib/Electrical Sources/Controlled Current Source  Initialize=on  Source_Type=AC  Amplitude=0  Phase=0  Frequency=0  Measurements=None
  Controlled Current Source1 : powerlib/Electrical Sources/Controlled Current Source  Initialize=on  Source_Type=AC  Amplitude=0  Phase=0  Frequency=0  Measurements=None
  Controlled Current Source2 : powerlib/Electrical Sources/Controlled Current Source  Initialize=on  Source_Type=AC  Amplitude=0  Phase=0  Frequency=0  Measurements=None
  Demux : Demux  Outputs=3
  Discrete-Time Integrator : DiscreteIntegrator  IntegratorMethod=Integration: Trapezoidal  InitialConditionSource=external  SampleTime=-1  ICPrevOutput=DiscIntNeverNeededParam  ICPrevScaledInput=DiscIntNeverNeededParam
  Gain : Gain  Gain=Wbase
  Gain1 : Gain  Gain=Sbase/Vbase
  Gain3 : Gain  Gain=1/Vbase
  Math Function1 : Math  Operator=mod  SignedPower=on  SaturateOnIntegerOverflow=on
  Mux : Mux  Inputs=3
  PQ Calculation (dq-Frame) : Subsystem  AncestorBlock=|
      | SimplusGT/PQ Calculation
      | (dq-Frame)
  Step : Step  Time=3  After=45/180*pi  SampleTime=Ts
  Sum : Sum  Inputs=|++
  Three-Phase Parallel RLC Branch : powerlib/Elements/Three-Phase Parallel RLC Branch  LConnTagsString=A|B|C  RConnTagsString=A|B|C  BranchType=C  Resistance=1  Inductance=1e-3  Capacitance=1e-9/Wbase*(Sbase/Vbase^2)  Measurements=None
      settings: SourceProductBaseCode=PS
  Voltage Measurement : powerlib/Measurements/Voltage Measurement  PhasorSimulation=off  OutputType=Complex  PSBequivalent=0
  Voltage Measurement1 : powerlib/Measurements/Voltage Measurement  PhasorSimulation=off  OutputType=Complex  PSBequivalent=0
  Voltage Measurement2 : powerlib/Measurements/Voltage Measurement  PhasorSimulation=off  OutputType=Complex  PSBequivalent=0
  "abc -> dq (Power-Invariant)" : Subsystem  AncestorBlock=|
      | SimplusGT/abc -> dq
      | (Power-Invariant)
  "dq -> abc (Power-Invariant)" : Subsystem  AncestorBlock=|
      | SimplusGT/dq -> abc
      | (Power-Invariant)
  a : PMIOPort  Side=Left
  b : PMIOPort  Port=2  Side=Left
  c : PMIOPort  Port=3  Side=Left
  n : PMIOPort  Port=4  Side=Left
  m : Outport
  wires:
  Gain/1 -> Discrete-Time Integrator/1
  Voltage Measurement2/1 -> Mux/3
  Voltage Measurement1/1 -> Mux/2
  Voltage Measurement/1 -> Mux/1
  [i_dq] -> PQ Calculation (dq-Frame)/2(idq)  "i_dq"
  [v_dq] -> PQ Calculation (dq-Frame)/1(vdq)  "v_dq"
  [v_abc] -> Bus Creator/3  "v_abc"
  Constant3/1 -> Math Function1/2
  [i_abc] -> Bus Creator/4  "i_abc"
  [theta] -> Bus Creator/6  "theta"
  Gain3/1 -> [v_abc]
  Constant2/1 -> Discrete-Time Integrator/2
  Math Function1/1 -> [theta], "dq -> abc (Power-Invariant)"/2(theta)
  Demux/1 -> Controlled Current Source/1
  Constant/1 -> [i_dq], "dq -> abc (Power-Invariant)"/1(dq)
  [i_abc] -> Gain1/1
  PQ Calculation (dq-Frame)/1(pq) -> [pq]
  [v_abc] -> "abc -> dq (Power-Invariant)"/1(abc)
  Mux/1 -> Gain3/1
  Gain1/1 -> Demux/1
  [w] -> Bus Creator/5  "w"
  [i_dq] -> Bus Creator/2  "i_dq"
  Constant1/1 -> [w], Gain/1
  Bus Creator/1 -> m/1
  "abc -> dq (Power-Invariant)"/1(dq) -> [v_dq]
  Demux/2 -> Controlled Current Source1/1
  [theta] -> "abc -> dq (Power-Invariant)"/2(theta)
  [pq] -> Bus Creator/7  "pq"
  "dq -> abc (Power-Invariant)"/1(abc) -> [i_abc]
  [v_dq] -> Bus Creator/1  "v_dq"
  Demux/3 -> Controlled Current Source2/1
  Sum/1 -> Math Function1/1
  Discrete-Time Integrator/1 -> Sum/1
  Step/1 -> Sum/2
  connections:
  Voltage Measurement/LConn1 -- Controlled Current Source/RConn1 -- Three-Phase Parallel RLC Branch/LConn1 -- a/RConn1
  Controlled Current Source/LConn1 -- Voltage Measurement/LConn2 -- Controlled Current Source1/LConn1 -- Voltage Measurement1/LConn2 -- Controlled Current Source2/LConn1 -- Voltage Measurement2/LConn2 -- Three-Phase Parallel RLC Branch/RConn2 -- Three-Phase Parallel RLC Branch/RConn3 -- Three-Phase Parallel RLC Branch/RConn1 -- n/RConn1
  Voltage Measurement2/LConn1 -- Controlled Current Source2/RConn1 -- Three-Phase Parallel RLC Branch/LConn3 -- c/RConn1
  Controlled Current Source1/RConn1 -- Voltage Measurement1/LConn1 -- Three-Phase Parallel RLC Branch/LConn2 -- b/RConn1

== system SingleInverterInfBus/AC Infinite Bus (Current Type)2 ==
  note: Electrical Circuit
  note: Auxiliary
  note: Current-type infinite bus.
      |
      | Author(s): Yitong Li
      |
      | Notes:
      |
      | Current-type means the infinite bus is a current source rather than a voltage source.
      |
      | The system is in source convention.
  Bus Creator : BusCreator  Inputs=7
  Constant : Constant  Value=[id iq]
  Constant1 : Constant  Value=w
  Constant2 : Constant  Value=theta0
  Constant3 : Constant  Value=2*pi
  Controlled Current Source : powerlib/Electrical Sources/Controlled Current Source  Initialize=on  Source_Type=AC  Amplitude=0  Phase=0  Frequency=0  Measurements=None
  Controlled Current Source1 : powerlib/Electrical Sources/Controlled Current Source  Initialize=on  Source_Type=AC  Amplitude=0  Phase=0  Frequency=0  Measurements=None
  Controlled Current Source2 : powerlib/Electrical Sources/Controlled Current Source  Initialize=on  Source_Type=AC  Amplitude=0  Phase=0  Frequency=0  Measurements=None
  Demux : Demux  Outputs=3
  Discrete-Time Integrator : DiscreteIntegrator  IntegratorMethod=Integration: Trapezoidal  InitialConditionSource=external  SampleTime=-1  ICPrevOutput=DiscIntNeverNeededParam  ICPrevScaledInput=DiscIntNeverNeededParam
  Gain : Gain  Gain=Wbase
  Gain1 : Gain  Gain=Sbase/Vbase
  Gain3 : Gain  Gain=1/Vbase
  Math Function1 : Math  Operator=mod  SignedPower=on  SaturateOnIntegerOverflow=on
  Mux : Mux  Inputs=3
  PQ Calculation (dq-Frame) : Subsystem  AncestorBlock=|
      | SimplusGT/PQ Calculation
      | (dq-Frame)
  Step : Step  Time=3  After=45/180*pi  SampleTime=Ts
  Sum : Sum  Inputs=|++
  Three-Phase Parallel RLC Branch : powerlib/Elements/Three-Phase Parallel RLC Branch  LConnTagsString=A|B|C  RConnTagsString=A|B|C  BranchType=C  Resistance=1  Inductance=1e-3  Capacitance=1e-9/Wbase*(Sbase/Vbase^2)  Measurements=None
      settings: SourceProductBaseCode=PS
  Voltage Measurement : powerlib/Measurements/Voltage Measurement  PhasorSimulation=off  OutputType=Complex  PSBequivalent=0
  Voltage Measurement1 : powerlib/Measurements/Voltage Measurement  PhasorSimulation=off  OutputType=Complex  PSBequivalent=0
  Voltage Measurement2 : powerlib/Measurements/Voltage Measurement  PhasorSimulation=off  OutputType=Complex  PSBequivalent=0
  "abc -> dq (Power-Invariant)" : Subsystem  AncestorBlock=|
      | SimplusGT/abc -> dq
      | (Power-Invariant)
  "dq -> abc (Power-Invariant)" : Subsystem  AncestorBlock=|
      | SimplusGT/dq -> abc
      | (Power-Invariant)
  a : PMIOPort  Side=Left
  b : PMIOPort  Port=2  Side=Left
  c : PMIOPort  Port=3  Side=Left
  n : PMIOPort  Port=4  Side=Left
  m : Outport
  wires:
  Gain/1 -> Discrete-Time Integrator/1
  Voltage Measurement2/1 -> Mux/3
  Voltage Measurement1/1 -> Mux/2
  Voltage Measurement/1 -> Mux/1
  [i_dq] -> PQ Calculation (dq-Frame)/2(idq)  "i_dq"
  [v_dq] -> PQ Calculation (dq-Frame)/1(vdq)  "v_dq"
  [v_abc] -> Bus Creator/3  "v_abc"
  Constant3/1 -> Math Function1/2
  [i_abc] -> Bus Creator/4  "i_abc"
  [theta] -> Bus Creator/6  "theta"
  Gain3/1 -> [v_abc]
  Constant2/1 -> Discrete-Time Integrator/2
  Math Function1/1 -> [theta], "dq -> abc (Power-Invariant)"/2(theta)
  Demux/1 -> Controlled Current Source/1
  Constant/1 -> [i_dq], "dq -> abc (Power-Invariant)"/1(dq)
  [i_abc] -> Gain1/1
  PQ Calculation (dq-Frame)/1(pq) -> [pq]
  [v_abc] -> "abc -> dq (Power-Invariant)"/1(abc)
  Mux/1 -> Gain3/1
  Gain1/1 -> Demux/1
  [w] -> Bus Creator/5  "w"
  [i_dq] -> Bus Creator/2  "i_dq"
  Constant1/1 -> [w], Gain/1
  Bus Creator/1 -> m/1
  "abc -> dq (Power-Invariant)"/1(dq) -> [v_dq]
  Demux/2 -> Controlled Current Source1/1
  [theta] -> "abc -> dq (Power-Invariant)"/2(theta)
  [pq] -> Bus Creator/7  "pq"
  "dq -> abc (Power-Invariant)"/1(abc) -> [i_abc]
  [v_dq] -> Bus Creator/1  "v_dq"
  Demux/3 -> Controlled Current Source2/1
  Sum/1 -> Math Function1/1
  Discrete-Time Integrator/1 -> Sum/1
  Step/1 -> Sum/2
  connections:
  Voltage Measurement/LConn1 -- Controlled Current Source/RConn1 -- Three-Phase Parallel RLC Branch/LConn1 -- a/RConn1
  Controlled Current Source/LConn1 -- Voltage Measurement/LConn2 -- Controlled Current Source1/LConn1 -- Voltage Measurement1/LConn2 -- Controlled Current Source2/LConn1 -- Voltage Measurement2/LConn2 -- Three-Phase Parallel RLC Branch/RConn2 -- Three-Phase Parallel RLC Branch/RConn3 -- Three-Phase Parallel RLC Branch/RConn1 -- n/RConn1
  Voltage Measurement2/LConn1 -- Controlled Current Source2/RConn1 -- Three-Phase Parallel RLC Branch/LConn3 -- c/RConn1
  Controlled Current Source1/RConn1 -- Voltage Measurement1/LConn1 -- Three-Phase Parallel RLC Branch/LConn2 -- b/RConn1

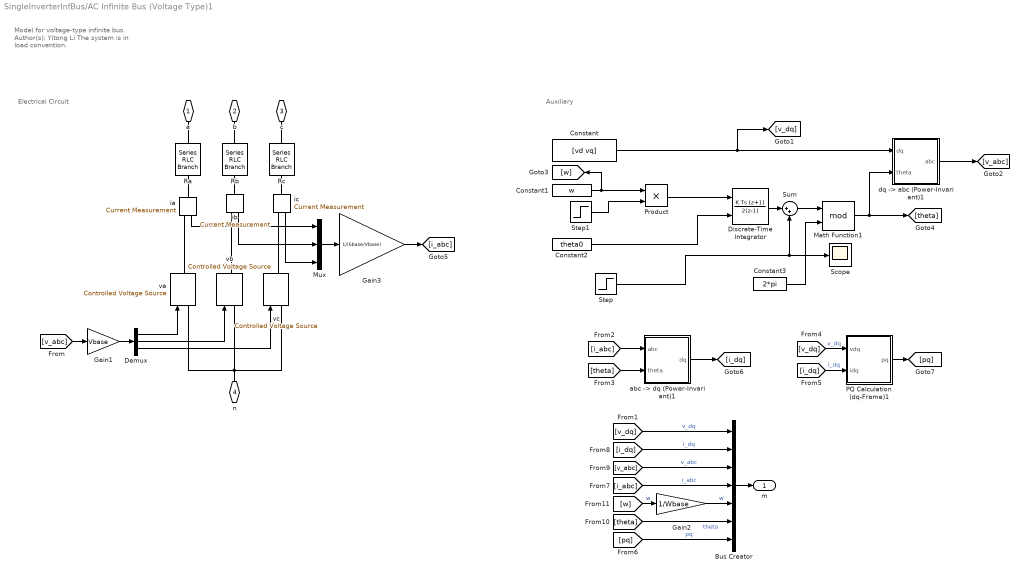
== system SingleInverterInfBus/AC Infinite Bus (Voltage Type)1 ==
  note: Auxiliary
  note: Electrical Circuit
  note: Model for voltage-type infinite bus.
      |
      | Author(s): Yitong Li
      |
      | The system is in load convention.
  Bus Creator : BusCreator  Inputs=7
  Constant : Constant  Value=[vd vq]
  Constant1 : Constant  Value=w
  Constant2 : Constant  Value=theta0
  Constant3 : Constant  Value=2*pi
  Demux : Demux  Outputs=3
  Discrete-Time Integrator : DiscreteIntegrator  IntegratorMethod=Integration: Trapezoidal  InitialConditionSource=external  SampleTime=-1  ICPrevOutput=DiscIntNeverNeededParam  ICPrevScaledInput=DiscIntNeverNeededParam
  Gain1 : Gain  Gain=Vbase
  Gain2 : Gain  Gain=1/Wbase
  Gain3 : Gain  Gain=1/(Sbase/Vbase)
  Math Function1 : Math  Operator=mod  SignedPower=on  SaturateOnIntegerOverflow=on
  Mux : Mux  Inputs=3
  PQ Calculation (dq-Frame)1 : Subsystem  AncestorBlock=|
      | SimplusGT/PQ Calculation
      | (dq-Frame)
  Product : Product
  Ra : powerlib/Elements/Series RLC Branch  LConnTagsString=__new0  RConnTagsString=__new0  BranchType=R  Resistance=R  Inductance=1e-3  SetiL0=off  InitialCurrent=0  Capacitance=1e-6  Setx0=off  InitialVoltage=0  Measurements=None
  Rb : powerlib/Elements/Series RLC Branch  LConnTagsString=__new0  RConnTagsString=__new0  BranchType=R  Resistance=R  Inductance=1e-3  SetiL0=off  InitialCurrent=0  Capacitance=1e-6  Setx0=off  InitialVoltage=0  Measurements=None
  Rc : powerlib/Elements/Series RLC Branch  LConnTagsString=__new0  RConnTagsString=__new0  BranchType=R  Resistance=R  Inductance=1e-3  SetiL0=off  InitialCurrent=0  Capacitance=1e-6  Setx0=off  InitialVoltage=0  Measurements=None
  Scope : Scope
  Step : Step  Time=3  After=45/180*pi  SampleTime=Ts
  Step1 : Step  Time=6  Before=1  After=0.99  SampleTime=Ts
  Sum : Sum  Inputs=|++
  "abc -> dq (Power-Invariant)1" : Subsystem  AncestorBlock=|
      | SimplusGT/abc -> dq
      | (Power-Invariant)
  "dq -> abc (Power-Invariant)1" : Subsystem  AncestorBlock=|
      | SimplusGT/dq -> abc
      | (Power-Invariant)
  ia : powerlib/Measurements/Current Measurement  PhasorSimulation=off  OutputType=Complex  PSBequivalent=0
  ib : powerlib/Measurements/Current Measurement  PhasorSimulation=off  OutputType=Complex  PSBequivalent=0
  ic : powerlib/Measurements/Current Measurement  PhasorSimulation=off  OutputType=Complex  PSBequivalent=0
  va : powerlib/Electrical Sources/Controlled Voltage Source  Initialize=on  Source_Type=AC  Amplitude=0  Phase=0  Frequency=0  Measurements=None
  vb : powerlib/Electrical Sources/Controlled Voltage Source  Initialize=on  Source_Type=AC  Amplitude=0  Phase=0  Frequency=0  Measurements=None
  vc : powerlib/Electrical Sources/Controlled Voltage Source  Initialize=on  Source_Type=AC  Amplitude=0  Phase=0  Frequency=0  Measurements=None
  a : PMIOPort  Side=Left
  b : PMIOPort  Port=2  Side=Left
  c : PMIOPort  Port=3  Side=Left
  n : PMIOPort  Port=4  Side=Left
  m : Outport
  wires:
  [pq] -> Bus Creator/7  "pq"
  PQ Calculation (dq-Frame)1/1(pq) -> [pq]
  [i_dq] -> PQ Calculation (dq-Frame)1/2(idq)  "i_dq"
  [v_dq] -> PQ Calculation (dq-Frame)1/1(vdq)  "v_dq"
  Gain3/1 -> [i_abc]
  Mux/1 -> Gain3/1
  Gain1/1 -> Demux/1
  "abc -> dq (Power-Invariant)1"/1(dq) -> [i_dq]
  [theta] -> "abc -> dq (Power-Invariant)1"/2(theta)
  [i_abc] -> "abc -> dq (Power-Invariant)1"/1(abc)
  ic/1 -> Mux/3
  ib/1 -> Mux/2
  ia/1 -> Mux/1
  [theta] -> Bus Creator/6  "theta"
  Bus Creator/1 -> m/1
  [i_dq] -> Bus Creator/2  "i_dq"
  Gain2/1 -> Bus Creator/5  "w"
  [v_abc] -> Bus Creator/3  "v_abc"
  [w] -> Gain2/1  "w"
  [i_abc] -> Bus Creator/4  "i_abc"
  [v_dq] -> Bus Creator/1  "v_dq"
  Constant/1 -> [v_dq], "dq -> abc (Power-Invariant)1"/1(dq)
  Constant3/1 -> Math Function1/2
  "dq -> abc (Power-Invariant)1"/1(abc) -> [v_abc]
  Constant1/1 -> Product/1, [w]
  Constant2/1 -> Discrete-Time Integrator/2
  Math Function1/1 -> [theta], "dq -> abc (Power-Invariant)1"/2(theta)
  Demux/3 -> vc/1
  Demux/2 -> vb/1
  Demux/1 -> va/1
  [v_abc] -> Gain1/1
  Discrete-Time Integrator/1 -> Sum/1
  Sum/1 -> Math Function1/1
  Step/1 -> Scope/1, Sum/2
  Product/1 -> Discrete-Time Integrator/1
  Step1/1 -> Product/2
  connections:
  Rc/LConn1 -- c/RConn1
  Rc/RConn1 -- ic/LConn1
  Rb/LConn1 -- b/RConn1
  ib/LConn1 -- Rb/RConn1
  Ra/LConn1 -- a/RConn1
  Ra/RConn1 -- ia/LConn1
  ic/RConn1 -- vc/RConn1
  ib/RConn1 -- vb/RConn1
  ia/RConn1 -- va/RConn1
  vb/LConn1 -- va/LConn1 -- n/RConn1 -- vc/LConn1

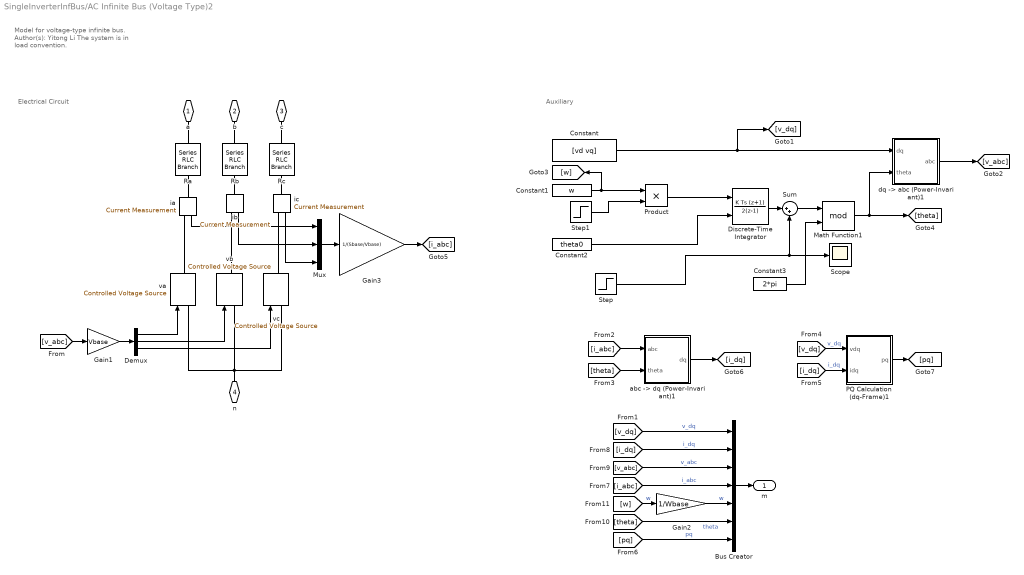
== system SingleInverterInfBus/AC Infinite Bus (Voltage Type)2 ==
  note: Auxiliary
  note: Electrical Circuit
  note: Model for voltage-type infinite bus.
      |
      | Author(s): Yitong Li
      |
      | The system is in load convention.
  Bus Creator : BusCreator  Inputs=7
  Constant : Constant  Value=[vd vq]
  Constant1 : Constant  Value=w
  Constant2 : Constant  Value=theta0
  Constant3 : Constant  Value=2*pi
  Demux : Demux  Outputs=3
  Discrete-Time Integrator : DiscreteIntegrator  IntegratorMethod=Integration: Trapezoidal  InitialConditionSource=external  SampleTime=-1  ICPrevOutput=DiscIntNeverNeededParam  ICPrevScaledInput=DiscIntNeverNeededParam
  Gain1 : Gain  Gain=Vbase
  Gain2 : Gain  Gain=1/Wbase
  Gain3 : Gain  Gain=1/(Sbase/Vbase)
  Math Function1 : Math  Operator=mod  SignedPower=on  SaturateOnIntegerOverflow=on
  Mux : Mux  Inputs=3
  PQ Calculation (dq-Frame)1 : Subsystem  AncestorBlock=|
      | SimplusGT/PQ Calculation
      | (dq-Frame)
  Product : Product
  Ra : powerlib/Elements/Series RLC Branch  LConnTagsString=__new0  RConnTagsString=__new0  BranchType=R  Resistance=R  Inductance=1e-3  SetiL0=off  InitialCurrent=0  Capacitance=1e-6  Setx0=off  InitialVoltage=0  Measurements=None
  Rb : powerlib/Elements/Series RLC Branch  LConnTagsString=__new0  RConnTagsString=__new0  BranchType=R  Resistance=R  Inductance=1e-3  SetiL0=off  InitialCurrent=0  Capacitance=1e-6  Setx0=off  InitialVoltage=0  Measurements=None
  Rc : powerlib/Elements/Series RLC Branch  LConnTagsString=__new0  RConnTagsString=__new0  BranchType=R  Resistance=R  Inductance=1e-3  SetiL0=off  InitialCurrent=0  Capacitance=1e-6  Setx0=off  InitialVoltage=0  Measurements=None
  Scope : Scope
  Step : Step  Time=3  After=45/180*pi  SampleTime=Ts
  Step1 : Step  Time=6  Before=1  After=0.99  SampleTime=Ts
  Sum : Sum  Inputs=|++
  "abc -> dq (Power-Invariant)1" : Subsystem  AncestorBlock=|
      | SimplusGT/abc -> dq
      | (Power-Invariant)
  "dq -> abc (Power-Invariant)1" : Subsystem  AncestorBlock=|
      | SimplusGT/dq -> abc
      | (Power-Invariant)
  ia : powerlib/Measurements/Current Measurement  PhasorSimulation=off  OutputType=Complex  PSBequivalent=0
  ib : powerlib/Measurements/Current Measurement  PhasorSimulation=off  OutputType=Complex  PSBequivalent=0
  ic : powerlib/Measurements/Current Measurement  PhasorSimulation=off  OutputType=Complex  PSBequivalent=0
  va : powerlib/Electrical Sources/Controlled Voltage Source  Initialize=on  Source_Type=AC  Amplitude=0  Phase=0  Frequency=0  Measurements=None
  vb : powerlib/Electrical Sources/Controlled Voltage Source  Initialize=on  Source_Type=AC  Amplitude=0  Phase=0  Frequency=0  Measurements=None
  vc : powerlib/Electrical Sources/Controlled Voltage Source  Initialize=on  Source_Type=AC  Amplitude=0  Phase=0  Frequency=0  Measurements=None
  a : PMIOPort  Side=Left
  b : PMIOPort  Port=2  Side=Left
  c : PMIOPort  Port=3  Side=Left
  n : PMIOPort  Port=4  Side=Left
  m : Outport
  wires:
  [pq] -> Bus Creator/7  "pq"
  PQ Calculation (dq-Frame)1/1(pq) -> [pq]
  [i_dq] -> PQ Calculation (dq-Frame)1/2(idq)  "i_dq"
  [v_dq] -> PQ Calculation (dq-Frame)1/1(vdq)  "v_dq"
  Gain3/1 -> [i_abc]
  Mux/1 -> Gain3/1
  Gain1/1 -> Demux/1
  "abc -> dq (Power-Invariant)1"/1(dq) -> [i_dq]
  [theta] -> "abc -> dq (Power-Invariant)1"/2(theta)
  [i_abc] -> "abc -> dq (Power-Invariant)1"/1(abc)
  ic/1 -> Mux/3
  ib/1 -> Mux/2
  ia/1 -> Mux/1
  [theta] -> Bus Creator/6  "theta"
  Bus Creator/1 -> m/1
  [i_dq] -> Bus Creator/2  "i_dq"
  Gain2/1 -> Bus Creator/5  "w"
  [v_abc] -> Bus Creator/3  "v_abc"
  [w] -> Gain2/1  "w"
  [i_abc] -> Bus Creator/4  "i_abc"
  [v_dq] -> Bus Creator/1  "v_dq"
  Constant/1 -> [v_dq], "dq -> abc (Power-Invariant)1"/1(dq)
  Constant3/1 -> Math Function1/2
  "dq -> abc (Power-Invariant)1"/1(abc) -> [v_abc]
  Constant1/1 -> Product/1, [w]
  Constant2/1 -> Discrete-Time Integrator/2
  Math Function1/1 -> [theta], "dq -> abc (Power-Invariant)1"/2(theta)
  Demux/3 -> vc/1
  Demux/2 -> vb/1
  Demux/1 -> va/1
  [v_abc] -> Gain1/1
  Discrete-Time Integrator/1 -> Sum/1
  Sum/1 -> Math Function1/1
  Step/1 -> Scope/1, Sum/2
  Product/1 -> Discrete-Time Integrator/1
  Step1/1 -> Product/2
  connections:
  Rc/LConn1 -- c/RConn1
  Rc/RConn1 -- ic/LConn1
  Rb/LConn1 -- b/RConn1
  ib/LConn1 -- Rb/RConn1
  Ra/LConn1 -- a/RConn1
  Ra/RConn1 -- ia/LConn1
  ic/RConn1 -- vc/RConn1
  ib/RConn1 -- vb/RConn1
  ia/RConn1 -- va/RConn1
  vb/LConn1 -- va/LConn1 -- n/RConn1 -- vc/LConn1
